simulink model "MOOD_DESLIZANTES"  (R2024a)
settings: Solver=VariableStepAuto  StartTime=0.0  StopTime=60  RelTol=1e-3
settings Model: Creator=VICTUS  LastModifiedBy=VICTUS

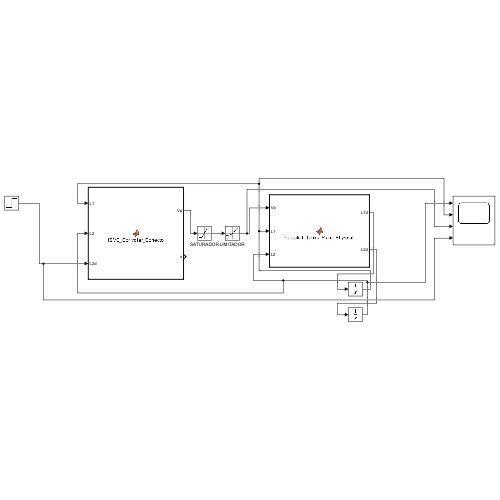
[thumbnail: Simulink's stored preview of the top-level diagram]
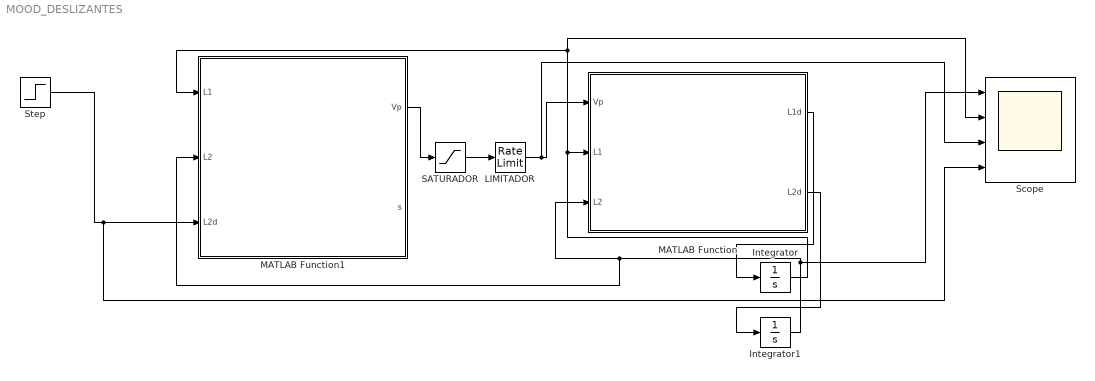
== system MOOD_DESLIZANTES ==
  Integrator : Integrator
  Integrator1 : Integrator
  LIMITADOR : RateLimiter  RisingSlewLimit=50  FallingSlewLimit=-50  SampleTimeMode=inherited
  MATLAB Function : MATLAB Function  TreatAsAtomicUnit=on
  MATLAB Function1 : MATLAB Function  TreatAsAtomicUnit=on
  SATURADOR : Saturate  UpperLimit=22  LowerLimit=0
  Scope : Scope  NumInputPorts=4
  Step : Step  Time=0  Before=0.01  After=10  SampleTime=0.01
  wires:
  MATLAB Function1/1(Vp) -> SATURADOR/1
  Step/1 -> Scope/4, MATLAB Function1/3(L2d)
  SATURADOR/1 -> LIMITADOR/1
  LIMITADOR/1 -> Scope/3, MATLAB Function/1(Vp)
  MATLAB Function/1(L1d) -> Integrator/1
  Integrator1/1 -> Scope/1, MATLAB Function1/2(L2), MATLAB Function/3(L2)
  MATLAB Function/2(L2d) -> Integrator1/1
  Integrator/1 -> Scope/2, MATLAB Function1/1(L1), MATLAB Function/2(L1)

== matlab function MOOD_DESLIZANTES/MATLAB Function1 ==
  settings: updateMethod=DISCRETE
  data: L1 input; Vp output; L2 input; L2d input; s output
function [Vp, s] = ISMC_Controller_Correcto(L1, L2, L2d)

%% ===== Estado persistente para el integrador =====
persistent e_int;
if isempty(e_int)
    e_int = 0; % Inicializar el integrador de error
end

%% ===== Parámetros físicos (Quanser) =====
dt1 = 4.445;   At1 = pi*(dt1^2)/4;
dt2 = 4.445;   At2 = pi*(dt2^2)/4;
d01 = 0.635;   Ao1 = pi*(d01^2)/4;
d02 = 0.47625; Ao2 = pi*(d02^2)/4;
Kp = 3.3;      g = 981;

k1 = Kp / At1;
k2 = (Ao1 * sqrt(2*g)) / At1;
k3 = (Ao1 * sqrt(2*g)) / At2;
k4 = (Ao2 * sqrt(2*g)) / At2;

%% ===== Parámetros de Sintonización =====
% ¡Estos valores son cruciales!
Ts = 0.01;      % ¡IMPORTANTE! Tiempo de muestreo (igual al de Simulink)

% Ganancias de la superficie (PID)
lambda1 = 6;  % Amortiguamiento (ajusta las oscilaciones)
lambda2 = 9;  % Acción integral (elimina error estacionario)

% Ganancias del control (SMC)
k = 0.5;        % Ganancia robusta (bajar si hay chattering)
phi = 0.1;      % Capa límite (subir si hay chattering)

%% ===== Protección de variables =====
L1 = max(L1, 1e-6);
L2 = max(L2, 1e-6);
%% ===== Cálculo de Errores y Superficie =====
e = L2 - L2d;                        % Error (e)
e_dot = (k3*sqrt(L1) - k4*sqrt(L2)); % Derivada del error (e_dot)

% Integrador (Euler)
e_int = e_int + e * Ts;

% Superficie de deslizamiento (s)
s = e_dot + lambda1 * e + lambda2 * e_int;


% Agrupando términos:
term_cancelacion = k2 * k3 / 2;
term_dinamica = (lambda1 - k4 / (2*sqrt(L2))) * e_dot;
term_integral = lambda2 * e;

% Función de saturación
sat_s = max(min(s/phi, 1), -1);
term_robusto = k * sat_s;

% Control calculado
Vp = (2*sqrt(L1) / (k1*k3)) * (term_cancelacion - term_dinamica - term_integral - term_robusto);

end

== matlab function MOOD_DESLIZANTES/MATLAB Function ==
  data: Vp input; L1d output; L2d output; L1 input; L2 input
function [L1d, L2d] = Coupled_Tanks_Plant_Physical(Vp,L1, L2)
% Modelo no lineal simplificado de tanques acoplados Quanser

dt1 = 4.445; dt2 = 4.445;
d01 = 0.635; d02 = 0.47625;
At1 = pi*(dt1^2)/4;  At2 = pi*(dt2^2)/4;
Ao1 = pi*(d01^2)/4;  Ao2 = pi*(d02^2)/4;
Kp = 3.3;  g = 981;


Fin = Kp * Vp;
Fout1 = Ao1 * sqrt(2*g*L1);
Fout2 = Ao2 * sqrt(2*g*L2);
F12 = Fout1;

L1d = (Fin - Fout1) / At1;
L2d = (F12 - Fout2) / At2;
end
